simulink model "linModel"  (R2024b)
settings: Solver=VariableStepAuto  StartTime=0.0  StopTime=60*4  RelTol=1e-3
values from neighbouring files (symbols this model uses):
  x0 = [85 ... (first row only)    [initConstants.m]
undefined symbols (not defined in the file or in its folder): A, B, C, D
settings Model: Creator=lahce  LastModifiedBy=lahce

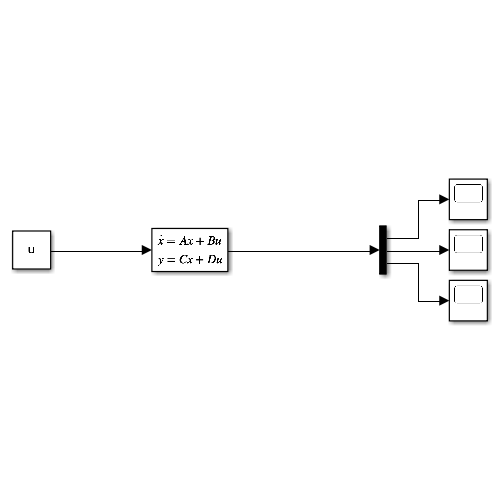
[thumbnail: Simulink's stored preview of the top-level diagram]
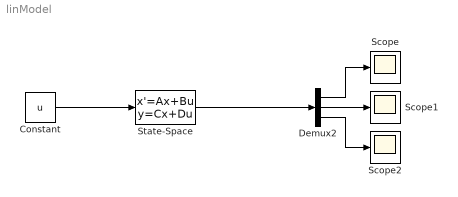
== system linModel ==
  Constant : Constant  Value=u
  Demux2 : Demux  Outputs=3
  Scope : Scope
  Scope1 : Scope
  Scope2 : Scope
  State-Space : StateSpace  A=A  B=B  C=C  D=D  InitialCondition=x0
  wires:
  Constant/1 -> State-Space/1
  Demux2/2 -> Scope1/1
  Demux2/1 -> Scope/1
  Demux2/3 -> Scope2/1
  State-Space/1 -> Demux2/1
